simulink model "inverted_pendulum_model_2018"  (R2018a)
settings: Solver=VariableStepAuto  StartTime=0.0  StopTime=10  RelTol=1e-3
values from neighbouring files (symbols this model uses):
  b = 0.1    [inverted_pendulum_parameter.m]
  g = 9.8    [inverted_pendulum_parameter.m]
  I = 0.0006    [inverted_pendulum_parameter.m]
  l = 0.3    [inverted_pendulum_parameter.m]
  M = 0.5    [inverted_pendulum_parameter.m]
  m = 0.2    [inverted_pendulum_parameter.m]
libraries: simulink x2
settings Model: Creator=Goku  LastModifiedBy=goku-ubuntu
settings DataIOCC: ReturnWorkspaceOutputs=on
settings SFSimCC: SimUseLocalCustomCode=on
settings RTWCC: RTWUseLocalCustomCode=on

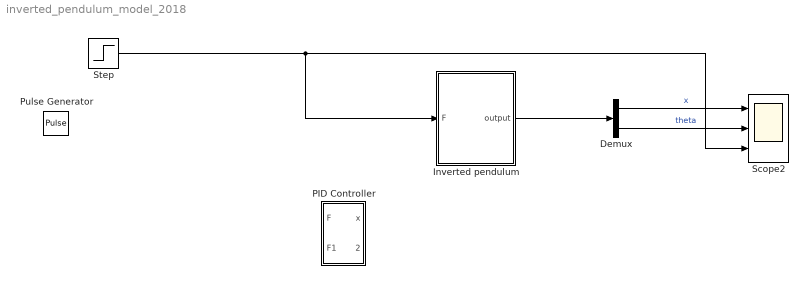
== system inverted_pendulum_model_2018 ==
  Demux : Demux  Outputs=2
  Inverted pendulum : Subsystem
  PID Controller : Subsystem
  Pulse Generator : DiscretePulseGenerator  PulseType=Time based  Amplitude=1000  Period=5  PulseWidth=.01
  Scope2 : Scope  NumInputPorts=3
  Step : Step  Time=0.01  Before=1  After=0  SampleTime=0
  wires:
  Demux/1 -> Scope2/1  "x"
  Demux/2 -> Scope2/2  "theta"
  Step/1 -> Scope2/3, Inverted pendulum/1(F)
  Inverted pendulum/1(output) -> Demux/1

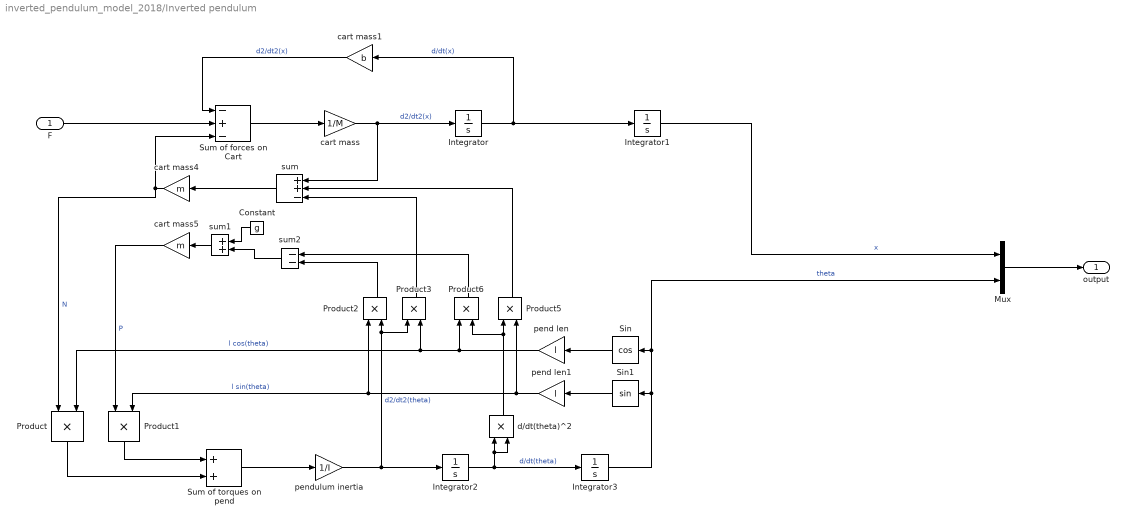
== system inverted_pendulum_model_2018/Inverted pendulum ==
  F : Inport
  Constant : Constant  Value=g
  Integrator{,1..3} (4 alike) : Integrator
  Mux : Mux  Inputs=2
  Product{,1..3,5..6} (6 alike) : Product
  Sin : Trigonometry  Operator=cos
  Sin1 : Trigonometry
  Sum of forces on Cart : Sum  Inputs=-+-
  Sum of torques on pend : Sum
  cart mass : Gain  Gain=1/M
  cart mass1 : Gain  Gain=b
  cart mass4 : Gain  Gain=m
  cart mass5 : Gain  Gain=m
  d/dt(theta)^2 : Product
  pend len : Gain  Gain=l
  pend len1 : Gain  Gain=l
  pendulum inertia : Gain  Gain=1/I
  sum : Sum  Inputs=++-
  sum1 : Sum
  sum2 : Sum  Inputs=--
  output : Outport  VectorParamsAs1DForOutWhenUnconnected=on
  wires:
  Mux/1 -> output/1
  Sum of forces on Cart/1 -> cart mass/1
  Integrator/1 -> cart mass1/1, Integrator1/1  "d/dt(x)"
  Product1/1 -> Sum of torques on pend/1
  Constant/1 -> sum1/1
  Integrator3/1 -> Mux/2, Sin/1, Sin1/1  "theta"
  cart mass5/1 -> Product1/1  "P"
  Product3/1 -> sum/3
  Integrator1/1 -> Mux/1  "x"
  cart mass1/1 -> Sum of forces on Cart/1  "d2/dt2(x)"
  Sin/1 -> pend len/1
  sum2/1 -> sum1/2
  cart mass4/1 -> Product/1, Sum of forces on Cart/3  "N"
  cart mass/1 -> sum/1, Integrator/1  "d2/dt2(x)"
  Sum of torques on pend/1 -> pendulum inertia/1
  Product6/1 -> sum2/1
  pendulum inertia/1 -> Product3/1, Product2/2, Integrator2/1  "d2/dt2(theta)"
  Product/1 -> Sum of torques on pend/2
  F/1 -> Sum of forces on Cart/2
  pend len/1 -> Product6/1, Product3/2, Product/2  "l cos(theta)"
  sum1/1 -> cart mass5/1
  Sin1/1 -> pend len1/1
  Product2/1 -> sum2/2
  d/dt(theta)^2/1 -> Product6/2, Product5/1
  sum/1 -> cart mass4/1
  pend len1/1 -> Product5/2, Product1/2, Product2/1  "l sin(theta)"
  Product5/1 -> sum/2
  Integrator2/1 -> Integrator3/1, d/dt(theta)^2/2, d/dt(theta)^2/1  "d/dt(theta)"

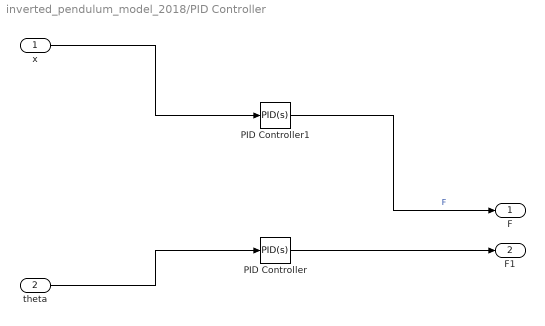
== system inverted_pendulum_model_2018/PID Controller ==
  x : Inport
  theta : Inport  Port=2
  PID Controller : simulink/Continuous/PID Controller  Controller=PID  TimeDomain=Continuous-time  SampleTime=-1  IntegratorMethod=Forward Euler  FilterMethod=Forward Euler  Form=Parallel  UseFilter=on  ControllerParametersSource=internal  P=1054.16123700867  I=2212.68658629558  D=61.4720921565294  N=100  InitialConditionSource=internal  InitialConditionForIntegrator=0  InitialConditionForFilter=0  ExternalReset=none  LimitOutput=off  UpperSaturationLimit=inf  LowerSaturationLimit=-inf  LinearizeAsGain=on  AntiWindupMode=none  Kb=1  TrackingMode=off  Kt=1  PParamMin=[]  PParamMax=[]  IParamMin=[]  IParamMax=[]  DParamMin=[]  DParamMax=[]  NParamMin=[]  NParamMax=[]  KbParamMin=[]  KbParamMax=[]  KtParamMin=[]  KtParamMax=[]  POutMin=[]  POutMax=[]  IOutMin=[]  IOutMax=[]  DOutMin=[]  DOutMax=[]  NOutMin=[]  NOutMax=[]  KbOutMin=[]  KbOutMax=[]  KtOutMin=[]  KtOutMax=[]  IntegratorOutMin=[]  IntegratorOutMax=[]  FilterOutMin=[]  FilterOutMax=[]  SumOutMin=[]  SumOutMax=[]  SumI1OutMin=[]  SumI1OutMax=[]  SumI2OutMin=[]  SumI2OutMax=[]  SumI3OutMin=[]  SumI3OutMax=[]  SumDOutMin=[]  SumDOutMax=[]  SaturationOutMin=[]  SaturationOutMax=[]  IntegratorContinuousStateAttributes=''  IntegratorStateMustResolveToSignalObject=off  IntegratorRTWStateStorageClass=Auto  FilterContinuousStateAttributes=''  FilterStateMustResolveToSignalObject=off  FilterRTWStateStorageClass=Auto  DifferentiatorICPrevScaledInput=0  DifferentiatorOutMin=[]  DifferentiatorOutMax=[]  FilterDiffOutCoefMin=[]  FilterDiffOutCoefMax=[]  SumDenOutMin=[]  SumDenOutMax=[]  SumNumOutMin=[]  SumNumOutMax=[]  ReciprocalOutMin=[]  ReciprocalOutMax=[]  DivideOutMin=[]  DivideOutMax=[]  TunerSelectOption=Transfer Function Based (PID Tuner App)
  PID Controller1 : simulink/Continuous/PID Controller  Controller=PID  TimeDomain=Continuous-time  SampleTime=-1  IntegratorMethod=Forward Euler  FilterMethod=Forward Euler  Form=Parallel  UseFilter=on  ControllerParametersSource=internal  P=-47.3373209436013  I=-1.83835720755632  D=23.1615902444953  N=0.356963663405428  InitialConditionSource=internal  InitialConditionForIntegrator=0  InitialConditionForFilter=0  ExternalReset=none  LimitOutput=off  UpperSaturationLimit=inf  LowerSaturationLimit=-inf  LinearizeAsGain=on  AntiWindupMode=none  Kb=1  TrackingMode=off  Kt=1  PParamMin=[]  PParamMax=[]  IParamMin=[]  IParamMax=[]  DParamMin=[]  DParamMax=[]  NParamMin=[]  NParamMax=[]  KbParamMin=[]  KbParamMax=[]  KtParamMin=[]  KtParamMax=[]  POutMin=[]  POutMax=[]  IOutMin=[]  IOutMax=[]  DOutMin=[]  DOutMax=[]  NOutMin=[]  NOutMax=[]  KbOutMin=[]  KbOutMax=[]  KtOutMin=[]  KtOutMax=[]  IntegratorOutMin=[]  IntegratorOutMax=[]  FilterOutMin=[]  FilterOutMax=[]  SumOutMin=[]  SumOutMax=[]  SumI1OutMin=[]  SumI1OutMax=[]  SumI2OutMin=[]  SumI2OutMax=[]  SumI3OutMin=[]  SumI3OutMax=[]  SumDOutMin=[]  SumDOutMax=[]  SaturationOutMin=[]  SaturationOutMax=[]  IntegratorContinuousStateAttributes=''  IntegratorStateMustResolveToSignalObject=off  IntegratorRTWStateStorageClass=Auto  FilterContinuousStateAttributes=''  FilterStateMustResolveToSignalObject=off  FilterRTWStateStorageClass=Auto  DifferentiatorICPrevScaledInput=0  DifferentiatorOutMin=[]  DifferentiatorOutMax=[]  FilterDiffOutCoefMin=[]  FilterDiffOutCoefMax=[]  SumDenOutMin=[]  SumDenOutMax=[]  SumNumOutMin=[]  SumNumOutMax=[]  ReciprocalOutMin=[]  ReciprocalOutMax=[]  DivideOutMin=[]  DivideOutMax=[]  TunerSelectOption=Transfer Function Based (PID Tuner App)
  F : Outport  VectorParamsAs1DForOutWhenUnconnected=on
  F1 : Outport  Port=2  VectorParamsAs1DForOutWhenUnconnected=on
  wires:
  PID Controller/1 -> F1/1
  theta/1 -> PID Controller/1
  PID Controller1/1 -> F/1  "F"
  x/1 -> PID Controller1/1
